simulink model "TST_EISGov_Governor"  (R2016b)
settings: Solver=FixedStepDiscrete  StartTime=0.0  StopTime=simTime  FixedStep=sampleTime  RelTol=1e-3
values from neighbouring files (symbols this model uses):
  testCase = 1    [initTST_EISGov_Governor_001.m]    (also in initTST_EISGov_Governor_002.m = 2; initTST_EISGov_Governor_003.m = 3; initTST_EISGov_Governor_004.m = 4; initTST_EISGov_Governor_005.m = 5)
libraries: simulink x43, UnitTest_Lib x36
(part 2 of 4)

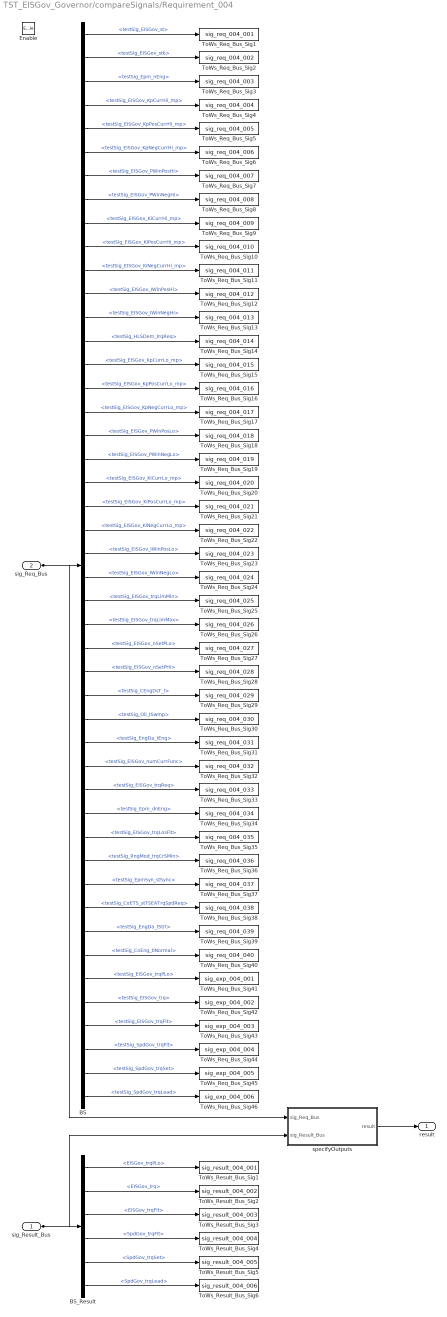
== system TST_EISGov_Governor/compareSignals/Requirement_004 ==
  sig_Result_Bus : Inport
  sig_Req_Bus : Inport  Port=2
  Enable : EnablePort
  BS : BusSelector  OutputSignals=testSig_EISGov_st,testSig_EISGov_st6,testSig_Epm_nEng,testSig_EISGov_KpCurrHi_mp,testSig_EISGov_KpPosCurrHi_mp,testSig_EISGov_KpNegCurrHi_mp,testSig_EISGov_PWinPosHi,testSig_EISGov_PWinNegHi,testSig_EISGov_KiCurrHi_mp,testSig_EISGov_KiPosCurrHi_mp,testSig_EISGov_KiNegCurrHi_mp,testSig_EISGov_IWinPosHi,testSig_EISGov_IWinNegHi,testSig_HLSDem_trqReq,testSig_EISGov_KpCurrLo_mp,testSig_EISGov_KpPosCurrLo_mp,testSig_EISGov_KpNegCurrLo_mp,testSig_EISGov_PWinPosLo,testSig_EISGov_PWinNegLo,testSig_EISGov_KiCurrLo_mp,testSig_EISGov_KiPosCurrLo_mp,testSig_EISGov_KiNegCurrLo_mp,testSig_EISGov_IWinPosLo,testSig_EISGov_IWinNegLo,testSig_EISGov_trqLimMin,testSig_EISGov_trqLimMax,testSig_EISGov_nSetPLo,testSig_EISGov_nSetPHi,testSig_CEngDsT_t,testSig_Oil_tSwmp,testSig_EngDa_tEng,testSig_EISGov_numCurrFunc,testSig_EISGov_trqReq,testSig_Epm_dnEng,testSig_EISGov_trqLosFlt,testSig_RngMod_trqCrSMin,testSig_EpmSyn_stSync,testSig_CoETS_stTSEATrqSpdReq,testSig_EngDa_tStrt,testSig_CoEng_tiNormal,testSig_EISGov_trqPLo,testSig_EISGov_trq,testSig_EISGov_trqFlt,testSig_SpdGov_trqFlt,testSig_SpdGov_trqSet,testSig_SpdGov_trqLead
  BS_Result : BusSelector  OutputSignals=EISGov_trqPLo,EISGov_trq,EISGov_trqFlt,SpdGov_trqFlt,SpdGov_trqSet,SpdGov_trqLead
  ToWs_Req_Bus_Sig1 : ToWorkspace  VariableName=sig_req_004_001  SaveFormat=Structure With Time
  ToWs_Req_Bus_Sig10 : ToWorkspace  VariableName=sig_req_004_010  SaveFormat=Structure With Time
  ToWs_Req_Bus_Sig11 : ToWorkspace  VariableName=sig_req_004_011  SaveFormat=Structure With Time
  ToWs_Req_Bus_Sig12 : ToWorkspace  VariableName=sig_req_004_012  SaveFormat=Structure With Time
  ToWs_Req_Bus_Sig13 : ToWorkspace  VariableName=sig_req_004_013  SaveFormat=Structure With Time
  ToWs_Req_Bus_Sig14 : ToWorkspace  VariableName=sig_req_004_014  SaveFormat=Structure With Time
  ToWs_Req_Bus_Sig15 : ToWorkspace  VariableName=sig_req_004_015  SaveFormat=Structure With Time
  ToWs_Req_Bus_Sig16 : ToWorkspace  VariableName=sig_req_004_016  SaveFormat=Structure With Time
  ToWs_Req_Bus_Sig17 : ToWorkspace  VariableName=sig_req_004_017  SaveFormat=Structure With Time
  ToWs_Req_Bus_Sig18 : ToWorkspace  VariableName=sig_req_004_018  SaveFormat=Structure With Time
  ToWs_Req_Bus_Sig19 : ToWorkspace  VariableName=sig_req_004_019  SaveFormat=Structure With Time
  ToWs_Req_Bus_Sig2 : ToWorkspace  VariableName=sig_req_004_002  SaveFormat=Structure With Time
  ToWs_Req_Bus_Sig20 : ToWorkspace  VariableName=sig_req_004_020  SaveFormat=Structure With Time
  ToWs_Req_Bus_Sig21 : ToWorkspace  VariableName=sig_req_004_021  SaveFormat=Structure With Time
  ToWs_Req_Bus_Sig22 : ToWorkspace  VariableName=sig_req_004_022  SaveFormat=Structure With Time
  ToWs_Req_Bus_Sig23 : ToWorkspace  VariableName=sig_req_004_023  SaveFormat=Structure With Time
  ToWs_Req_Bus_Sig24 : ToWorkspace  VariableName=sig_req_004_024  SaveFormat=Structure With Time
  ToWs_Req_Bus_Sig25 : ToWorkspace  VariableName=sig_req_004_025  SaveFormat=Structure With Time
  ToWs_Req_Bus_Sig26 : ToWorkspace  VariableName=sig_req_004_026  SaveFormat=Structure With Time
  ToWs_Req_Bus_Sig27 : ToWorkspace  VariableName=sig_req_004_027  SaveFormat=Structure With Time
  ToWs_Req_Bus_Sig28 : ToWorkspace  VariableName=sig_req_004_028  SaveFormat=Structure With Time
  ToWs_Req_Bus_Sig29 : ToWorkspace  VariableName=sig_req_004_029  SaveFormat=Structure With Time
  ToWs_Req_Bus_Sig3 : ToWorkspace  VariableName=sig_req_004_003  SaveFormat=Structure With Time
  ToWs_Req_Bus_Sig30 : ToWorkspace  VariableName=sig_req_004_030  SaveFormat=Structure With Time
  ToWs_Req_Bus_Sig31 : ToWorkspace  VariableName=sig_req_004_031  SaveFormat=Structure With Time
  ToWs_Req_Bus_Sig32 : ToWorkspace  VariableName=sig_req_004_032  SaveFormat=Structure With Time
  ToWs_Req_Bus_Sig33 : ToWorkspace  VariableName=sig_req_004_033  SaveFormat=Structure With Time
  ToWs_Req_Bus_Sig34 : ToWorkspace  VariableName=sig_req_004_034  SaveFormat=Structure With Time
  ToWs_Req_Bus_Sig35 : ToWorkspace  VariableName=sig_req_004_035  SaveFormat=Structure With Time
  ToWs_Req_Bus_Sig36 : ToWorkspace  VariableName=sig_req_004_036  SaveFormat=Structure With Time
  ToWs_Req_Bus_Sig37 : ToWorkspace  VariableName=sig_req_004_037  SaveFormat=Structure With Time
  ToWs_Req_Bus_Sig38 : ToWorkspace  VariableName=sig_req_004_038  SaveFormat=Structure With Time
  ToWs_Req_Bus_Sig39 : ToWorkspace  VariableName=sig_req_004_039  SaveFormat=Structure With Time
  ToWs_Req_Bus_Sig4 : ToWorkspace  VariableName=sig_req_004_004  SaveFormat=Structure With Time
  ToWs_Req_Bus_Sig40 : ToWorkspace  VariableName=sig_req_004_040  SaveFormat=Structure With Time
  ToWs_Req_Bus_Sig41 : ToWorkspace  VariableName=sig_exp_004_001  SaveFormat=Structure With Time
  ToWs_Req_Bus_Sig42 : ToWorkspace  VariableName=sig_exp_004_002  SaveFormat=Structure With Time
  ToWs_Req_Bus_Sig43 : ToWorkspace  VariableName=sig_exp_004_003  SaveFormat=Structure With Time
  ToWs_Req_Bus_Sig44 : ToWorkspace  VariableName=sig_exp_004_004  SaveFormat=Structure With Time
  ToWs_Req_Bus_Sig45 : ToWorkspace  VariableName=sig_exp_004_005  SaveFormat=Structure With Time
  ToWs_Req_Bus_Sig46 : ToWorkspace  VariableName=sig_exp_004_006  SaveFormat=Structure With Time
  ToWs_Req_Bus_Sig5 : ToWorkspace  VariableName=sig_req_004_005  SaveFormat=Structure With Time
  ToWs_Req_Bus_Sig6 : ToWorkspace  VariableName=sig_req_004_006  SaveFormat=Structure With Time
  ToWs_Req_Bus_Sig7 : ToWorkspace  VariableName=sig_req_004_007  SaveFormat=Structure With Time
  ToWs_Req_Bus_Sig8 : ToWorkspace  VariableName=sig_req_004_008  SaveFormat=Structure With Time
  ToWs_Req_Bus_Sig9 : ToWorkspace  VariableName=sig_req_004_009  SaveFormat=Structure With Time
  ToWs_Result_Bus_Sig1 : ToWorkspace  VariableName=sig_result_004_001  SaveFormat=Structure With Time
  ToWs_Result_Bus_Sig2 : ToWorkspace  VariableName=sig_result_004_002  SaveFormat=Structure With Time
  ToWs_Result_Bus_Sig3 : ToWorkspace  VariableName=sig_result_004_003  SaveFormat=Structure With Time
  ToWs_Result_Bus_Sig4 : ToWorkspace  VariableName=sig_result_004_004  SaveFormat=Structure With Time
  ToWs_Result_Bus_Sig5 : ToWorkspace  VariableName=sig_result_004_005  SaveFormat=Structure With Time
  ToWs_Result_Bus_Sig6 : ToWorkspace  VariableName=sig_result_004_006  SaveFormat=Structure With Time
  specifyOutputs : Subsystem
  result : Outport
  wires:
  sig_Req_Bus/1 -> BS/1, specifyOutputs/1(sig_Req_Bus)
  BS/1 -> ToWs_Req_Bus_Sig1/1  "<testSig_EISGov_st>"
  BS/2 -> ToWs_Req_Bus_Sig2/1  "<testSig_EISGov_st6>"
  BS/3 -> ToWs_Req_Bus_Sig3/1  "<testSig_Epm_nEng>"
  BS/4 -> ToWs_Req_Bus_Sig4/1  "<testSig_EISGov_KpCurrHi_mp>"
  BS/5 -> ToWs_Req_Bus_Sig5/1  "<testSig_EISGov_KpPosCurrHi_mp>"
  BS/6 -> ToWs_Req_Bus_Sig6/1  "<testSig_EISGov_KpNegCurrHi_mp>"
  BS/7 -> ToWs_Req_Bus_Sig7/1  "<testSig_EISGov_PWinPosHi>"
  BS/8 -> ToWs_Req_Bus_Sig8/1  "<testSig_EISGov_PWinNegHi>"
  BS/9 -> ToWs_Req_Bus_Sig9/1  "<testSig_EISGov_KiCurrHi_mp>"
  BS/10 -> ToWs_Req_Bus_Sig10/1  "<testSig_EISGov_KiPosCurrHi_mp>"
  BS/11 -> ToWs_Req_Bus_Sig11/1  "<testSig_EISGov_KiNegCurrHi_mp>"
  BS/12 -> ToWs_Req_Bus_Sig12/1  "<testSig_EISGov_IWinPosHi>"
  BS/13 -> ToWs_Req_Bus_Sig13/1  "<testSig_EISGov_IWinNegHi>"
  BS/14 -> ToWs_Req_Bus_Sig14/1  "<testSig_HLSDem_trqReq>"
  BS/15 -> ToWs_Req_Bus_Sig15/1  "<testSig_EISGov_KpCurrLo_mp>"
  BS/16 -> ToWs_Req_Bus_Sig16/1  "<testSig_EISGov_KpPosCurrLo_mp>"
  BS/17 -> ToWs_Req_Bus_Sig17/1  "<testSig_EISGov_KpNegCurrLo_mp>"
  BS/18 -> ToWs_Req_Bus_Sig18/1  "<testSig_EISGov_PWinPosLo>"
  BS/19 -> ToWs_Req_Bus_Sig19/1  "<testSig_EISGov_PWinNegLo>"
  BS/20 -> ToWs_Req_Bus_Sig20/1  "<testSig_EISGov_KiCurrLo_mp>"
  BS/21 -> ToWs_Req_Bus_Sig21/1  "<testSig_EISGov_KiPosCurrLo_mp>"
  BS/22 -> ToWs_Req_Bus_Sig22/1  "<testSig_EISGov_KiNegCurrLo_mp>"
  BS/23 -> ToWs_Req_Bus_Sig23/1  "<testSig_EISGov_IWinPosLo>"
  BS/24 -> ToWs_Req_Bus_Sig24/1  "<testSig_EISGov_IWinNegLo>"
  BS/25 -> ToWs_Req_Bus_Sig25/1  "<testSig_EISGov_trqLimMin>"
  BS/26 -> ToWs_Req_Bus_Sig26/1  "<testSig_EISGov_trqLimMax>"
  BS/27 -> ToWs_Req_Bus_Sig27/1  "<testSig_EISGov_nSetPLo>"
  BS/28 -> ToWs_Req_Bus_Sig28/1  "<testSig_EISGov_nSetPHi>"
  BS/29 -> ToWs_Req_Bus_Sig29/1  "<testSig_CEngDsT_t>"
  BS/30 -> ToWs_Req_Bus_Sig30/1  "<testSig_Oil_tSwmp>"
  BS/31 -> ToWs_Req_Bus_Sig31/1  "<testSig_EngDa_tEng>"
  BS/32 -> ToWs_Req_Bus_Sig32/1  "<testSig_EISGov_numCurrFunc>"
  BS/33 -> ToWs_Req_Bus_Sig33/1  "<testSig_EISGov_trqReq>"
  BS/34 -> ToWs_Req_Bus_Sig34/1  "<testSig_Epm_dnEng>"
  BS/35 -> ToWs_Req_Bus_Sig35/1  "<testSig_EISGov_trqLosFlt>"
  BS/36 -> ToWs_Req_Bus_Sig36/1  "<testSig_RngMod_trqCrSMin>"
  BS/37 -> ToWs_Req_Bus_Sig37/1  "<testSig_EpmSyn_stSync>"
  BS/38 -> ToWs_Req_Bus_Sig38/1  "<testSig_CoETS_stTSEATrqSpdReq>"
  BS/39 -> ToWs_Req_Bus_Sig39/1  "<testSig_EngDa_tStrt>"
  BS/40 -> ToWs_Req_Bus_Sig40/1  "<testSig_CoEng_tiNormal>"
  BS/41 -> ToWs_Req_Bus_Sig41/1  "<testSig_EISGov_trqPLo>"
  BS/42 -> ToWs_Req_Bus_Sig42/1  "<testSig_EISGov_trq>"
  BS/43 -> ToWs_Req_Bus_Sig43/1  "<testSig_EISGov_trqFlt>"
  BS/44 -> ToWs_Req_Bus_Sig44/1  "<testSig_SpdGov_trqFlt>"
  BS/45 -> ToWs_Req_Bus_Sig45/1  "<testSig_SpdGov_trqSet>"
  BS/46 -> ToWs_Req_Bus_Sig46/1  "<testSig_SpdGov_trqLead>"
  sig_Result_Bus/1 -> BS_Result/1, specifyOutputs/2(sig_Result_Bus)
  BS_Result/1 -> ToWs_Result_Bus_Sig1/1  "<EISGov_trqPLo>"
  BS_Result/2 -> ToWs_Result_Bus_Sig2/1  "<EISGov_trq>"
  BS_Result/3 -> ToWs_Result_Bus_Sig3/1  "<EISGov_trqFlt>"
  BS_Result/4 -> ToWs_Result_Bus_Sig4/1  "<SpdGov_trqFlt>"
  BS_Result/5 -> ToWs_Result_Bus_Sig5/1  "<SpdGov_trqSet>"
  BS_Result/6 -> ToWs_Result_Bus_Sig6/1  "<SpdGov_trqLead>"
  specifyOutputs/1(result) -> result/1

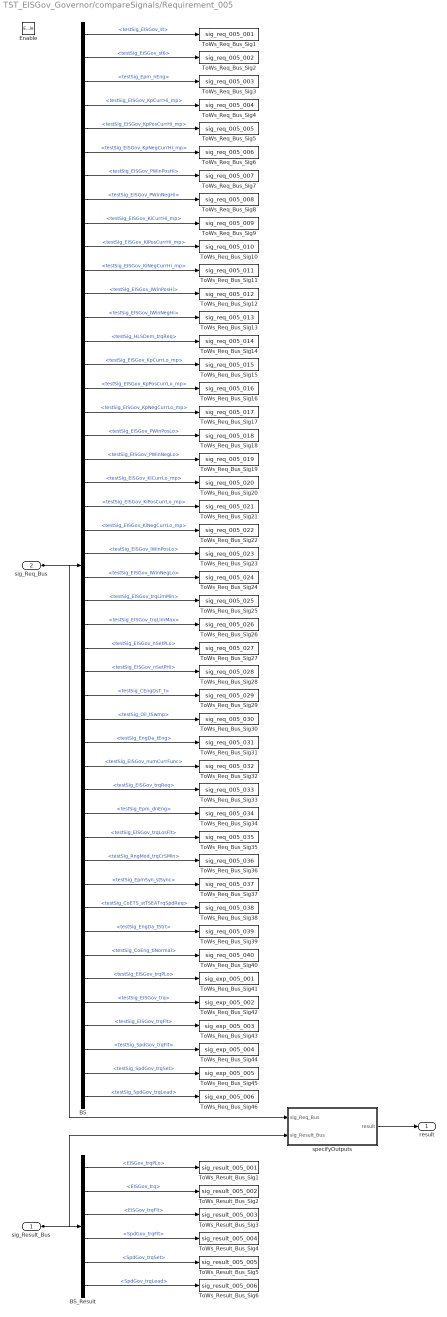
== system TST_EISGov_Governor/compareSignals/Requirement_005 ==
  sig_Result_Bus : Inport
  sig_Req_Bus : Inport  Port=2
  Enable : EnablePort
  BS : BusSelector  OutputSignals=testSig_EISGov_st,testSig_EISGov_st6,testSig_Epm_nEng,testSig_EISGov_KpCurrHi_mp,testSig_EISGov_KpPosCurrHi_mp,testSig_EISGov_KpNegCurrHi_mp,testSig_EISGov_PWinPosHi,testSig_EISGov_PWinNegHi,testSig_EISGov_KiCurrHi_mp,testSig_EISGov_KiPosCurrHi_mp,testSig_EISGov_KiNegCurrHi_mp,testSig_EISGov_IWinPosHi,testSig_EISGov_IWinNegHi,testSig_HLSDem_trqReq,testSig_EISGov_KpCurrLo_mp,testSig_EISGov_KpPosCurrLo_mp,testSig_EISGov_KpNegCurrLo_mp,testSig_EISGov_PWinPosLo,testSig_EISGov_PWinNegLo,testSig_EISGov_KiCurrLo_mp,testSig_EISGov_KiPosCurrLo_mp,testSig_EISGov_KiNegCurrLo_mp,testSig_EISGov_IWinPosLo,testSig_EISGov_IWinNegLo,testSig_EISGov_trqLimMin,testSig_EISGov_trqLimMax,testSig_EISGov_nSetPLo,testSig_EISGov_nSetPHi,testSig_CEngDsT_t,testSig_Oil_tSwmp,testSig_EngDa_tEng,testSig_EISGov_numCurrFunc,testSig_EISGov_trqReq,testSig_Epm_dnEng,testSig_EISGov_trqLosFlt,testSig_RngMod_trqCrSMin,testSig_EpmSyn_stSync,testSig_CoETS_stTSEATrqSpdReq,testSig_EngDa_tStrt,testSig_CoEng_tiNormal,testSig_EISGov_trqPLo,testSig_EISGov_trq,testSig_EISGov_trqFlt,testSig_SpdGov_trqFlt,testSig_SpdGov_trqSet,testSig_SpdGov_trqLead
  BS_Result : BusSelector  OutputSignals=EISGov_trqPLo,EISGov_trq,EISGov_trqFlt,SpdGov_trqFlt,SpdGov_trqSet,SpdGov_trqLead
  ToWs_Req_Bus_Sig1 : ToWorkspace  VariableName=sig_req_005_001  SaveFormat=Structure With Time
  ToWs_Req_Bus_Sig10 : ToWorkspace  VariableName=sig_req_005_010  SaveFormat=Structure With Time
  ToWs_Req_Bus_Sig11 : ToWorkspace  VariableName=sig_req_005_011  SaveFormat=Structure With Time
  ToWs_Req_Bus_Sig12 : ToWorkspace  VariableName=sig_req_005_012  SaveFormat=Structure With Time
  ToWs_Req_Bus_Sig13 : ToWorkspace  VariableName=sig_req_005_013  SaveFormat=Structure With Time
  ToWs_Req_Bus_Sig14 : ToWorkspace  VariableName=sig_req_005_014  SaveFormat=Structure With Time
  ToWs_Req_Bus_Sig15 : ToWorkspace  VariableName=sig_req_005_015  SaveFormat=Structure With Time
  ToWs_Req_Bus_Sig16 : ToWorkspace  VariableName=sig_req_005_016  SaveFormat=Structure With Time
  ToWs_Req_Bus_Sig17 : ToWorkspace  VariableName=sig_req_005_017  SaveFormat=Structure With Time
  ToWs_Req_Bus_Sig18 : ToWorkspace  VariableName=sig_req_005_018  SaveFormat=Structure With Time
  ToWs_Req_Bus_Sig19 : ToWorkspace  VariableName=sig_req_005_019  SaveFormat=Structure With Time
  ToWs_Req_Bus_Sig2 : ToWorkspace  VariableName=sig_req_005_002  SaveFormat=Structure With Time
  ToWs_Req_Bus_Sig20 : ToWorkspace  VariableName=sig_req_005_020  SaveFormat=Structure With Time
  ToWs_Req_Bus_Sig21 : ToWorkspace  VariableName=sig_req_005_021  SaveFormat=Structure With Time
  ToWs_Req_Bus_Sig22 : ToWorkspace  VariableName=sig_req_005_022  SaveFormat=Structure With Time
  ToWs_Req_Bus_Sig23 : ToWorkspace  VariableName=sig_req_005_023  SaveFormat=Structure With Time
  ToWs_Req_Bus_Sig24 : ToWorkspace  VariableName=sig_req_005_024  SaveFormat=Structure With Time
  ToWs_Req_Bus_Sig25 : ToWorkspace  VariableName=sig_req_005_025  SaveFormat=Structure With Time
  ToWs_Req_Bus_Sig26 : ToWorkspace  VariableName=sig_req_005_026  SaveFormat=Structure With Time
  ToWs_Req_Bus_Sig27 : ToWorkspace  VariableName=sig_req_005_027  SaveFormat=Structure With Time
  ToWs_Req_Bus_Sig28 : ToWorkspace  VariableName=sig_req_005_028  SaveFormat=Structure With Time
  ToWs_Req_Bus_Sig29 : ToWorkspace  VariableName=sig_req_005_029  SaveFormat=Structure With Time
  ToWs_Req_Bus_Sig3 : ToWorkspace  VariableName=sig_req_005_003  SaveFormat=Structure With Time
  ToWs_Req_Bus_Sig30 : ToWorkspace  VariableName=sig_req_005_030  SaveFormat=Structure With Time
  ToWs_Req_Bus_Sig31 : ToWorkspace  VariableName=sig_req_005_031  SaveFormat=Structure With Time
  ToWs_Req_Bus_Sig32 : ToWorkspace  VariableName=sig_req_005_032  SaveFormat=Structure With Time
  ToWs_Req_Bus_Sig33 : ToWorkspace  VariableName=sig_req_005_033  SaveFormat=Structure With Time
  ToWs_Req_Bus_Sig34 : ToWorkspace  VariableName=sig_req_005_034  SaveFormat=Structure With Time
  ToWs_Req_Bus_Sig35 : ToWorkspace  VariableName=sig_req_005_035  SaveFormat=Structure With Time
  ToWs_Req_Bus_Sig36 : ToWorkspace  VariableName=sig_req_005_036  SaveFormat=Structure With Time
  ToWs_Req_Bus_Sig37 : ToWorkspace  VariableName=sig_req_005_037  SaveFormat=Structure With Time
  ToWs_Req_Bus_Sig38 : ToWorkspace  VariableName=sig_req_005_038  SaveFormat=Structure With Time
  ToWs_Req_Bus_Sig39 : ToWorkspace  VariableName=sig_req_005_039  SaveFormat=Structure With Time
  ToWs_Req_Bus_Sig4 : ToWorkspace  VariableName=sig_req_005_004  SaveFormat=Structure With Time
  ToWs_Req_Bus_Sig40 : ToWorkspace  VariableName=sig_req_005_040  SaveFormat=Structure With Time
  ToWs_Req_Bus_Sig41 : ToWorkspace  VariableName=sig_exp_005_001  SaveFormat=Structure With Time
  ToWs_Req_Bus_Sig42 : ToWorkspace  VariableName=sig_exp_005_002  SaveFormat=Structure With Time
  ToWs_Req_Bus_Sig43 : ToWorkspace  VariableName=sig_exp_005_003  SaveFormat=Structure With Time
  ToWs_Req_Bus_Sig44 : ToWorkspace  VariableName=sig_exp_005_004  SaveFormat=Structure With Time
  ToWs_Req_Bus_Sig45 : ToWorkspace  VariableName=sig_exp_005_005  SaveFormat=Structure With Time
  ToWs_Req_Bus_Sig46 : ToWorkspace  VariableName=sig_exp_005_006  SaveFormat=Structure With Time
  ToWs_Req_Bus_Sig5 : ToWorkspace  VariableName=sig_req_005_005  SaveFormat=Structure With Time
  ToWs_Req_Bus_Sig6 : ToWorkspace  VariableName=sig_req_005_006  SaveFormat=Structure With Time
  ToWs_Req_Bus_Sig7 : ToWorkspace  VariableName=sig_req_005_007  SaveFormat=Structure With Time
  ToWs_Req_Bus_Sig8 : ToWorkspace  VariableName=sig_req_005_008  SaveFormat=Structure With Time
  ToWs_Req_Bus_Sig9 : ToWorkspace  VariableName=sig_req_005_009  SaveFormat=Structure With Time
  ToWs_Result_Bus_Sig1 : ToWorkspace  VariableName=sig_result_005_001  SaveFormat=Structure With Time
  ToWs_Result_Bus_Sig2 : ToWorkspace  VariableName=sig_result_005_002  SaveFormat=Structure With Time
  ToWs_Result_Bus_Sig3 : ToWorkspace  VariableName=sig_result_005_003  SaveFormat=Structure With Time
  ToWs_Result_Bus_Sig4 : ToWorkspace  VariableName=sig_result_005_004  SaveFormat=Structure With Time
  ToWs_Result_Bus_Sig5 : ToWorkspace  VariableName=sig_result_005_005  SaveFormat=Structure With Time
  ToWs_Result_Bus_Sig6 : ToWorkspace  VariableName=sig_result_005_006  SaveFormat=Structure With Time
  specifyOutputs : Subsystem
  result : Outport
  wires:
  sig_Req_Bus/1 -> BS/1, specifyOutputs/1(sig_Req_Bus)
  BS/1 -> ToWs_Req_Bus_Sig1/1  "<testSig_EISGov_st>"
  BS/2 -> ToWs_Req_Bus_Sig2/1  "<testSig_EISGov_st6>"
  BS/3 -> ToWs_Req_Bus_Sig3/1  "<testSig_Epm_nEng>"
  BS/4 -> ToWs_Req_Bus_Sig4/1  "<testSig_EISGov_KpCurrHi_mp>"
  BS/5 -> ToWs_Req_Bus_Sig5/1  "<testSig_EISGov_KpPosCurrHi_mp>"
  BS/6 -> ToWs_Req_Bus_Sig6/1  "<testSig_EISGov_KpNegCurrHi_mp>"
  BS/7 -> ToWs_Req_Bus_Sig7/1  "<testSig_EISGov_PWinPosHi>"
  BS/8 -> ToWs_Req_Bus_Sig8/1  "<testSig_EISGov_PWinNegHi>"
  BS/9 -> ToWs_Req_Bus_Sig9/1  "<testSig_EISGov_KiCurrHi_mp>"
  BS/10 -> ToWs_Req_Bus_Sig10/1  "<testSig_EISGov_KiPosCurrHi_mp>"
  BS/11 -> ToWs_Req_Bus_Sig11/1  "<testSig_EISGov_KiNegCurrHi_mp>"
  BS/12 -> ToWs_Req_Bus_Sig12/1  "<testSig_EISGov_IWinPosHi>"
  BS/13 -> ToWs_Req_Bus_Sig13/1  "<testSig_EISGov_IWinNegHi>"
  BS/14 -> ToWs_Req_Bus_Sig14/1  "<testSig_HLSDem_trqReq>"
  BS/15 -> ToWs_Req_Bus_Sig15/1  "<testSig_EISGov_KpCurrLo_mp>"
  BS/16 -> ToWs_Req_Bus_Sig16/1  "<testSig_EISGov_KpPosCurrLo_mp>"
  BS/17 -> ToWs_Req_Bus_Sig17/1  "<testSig_EISGov_KpNegCurrLo_mp>"
  BS/18 -> ToWs_Req_Bus_Sig18/1  "<testSig_EISGov_PWinPosLo>"
  BS/19 -> ToWs_Req_Bus_Sig19/1  "<testSig_EISGov_PWinNegLo>"
  BS/20 -> ToWs_Req_Bus_Sig20/1  "<testSig_EISGov_KiCurrLo_mp>"
  BS/21 -> ToWs_Req_Bus_Sig21/1  "<testSig_EISGov_KiPosCurrLo_mp>"
  BS/22 -> ToWs_Req_Bus_Sig22/1  "<testSig_EISGov_KiNegCurrLo_mp>"
  BS/23 -> ToWs_Req_Bus_Sig23/1  "<testSig_EISGov_IWinPosLo>"
  BS/24 -> ToWs_Req_Bus_Sig24/1  "<testSig_EISGov_IWinNegLo>"
  BS/25 -> ToWs_Req_Bus_Sig25/1  "<testSig_EISGov_trqLimMin>"
  BS/26 -> ToWs_Req_Bus_Sig26/1  "<testSig_EISGov_trqLimMax>"
  BS/27 -> ToWs_Req_Bus_Sig27/1  "<testSig_EISGov_nSetPLo>"
  BS/28 -> ToWs_Req_Bus_Sig28/1  "<testSig_EISGov_nSetPHi>"
  BS/29 -> ToWs_Req_Bus_Sig29/1  "<testSig_CEngDsT_t>"
  BS/30 -> ToWs_Req_Bus_Sig30/1  "<testSig_Oil_tSwmp>"
  BS/31 -> ToWs_Req_Bus_Sig31/1  "<testSig_EngDa_tEng>"
  BS/32 -> ToWs_Req_Bus_Sig32/1  "<testSig_EISGov_numCurrFunc>"
  BS/33 -> ToWs_Req_Bus_Sig33/1  "<testSig_EISGov_trqReq>"
  BS/34 -> ToWs_Req_Bus_Sig34/1  "<testSig_Epm_dnEng>"
  BS/35 -> ToWs_Req_Bus_Sig35/1  "<testSig_EISGov_trqLosFlt>"
  BS/36 -> ToWs_Req_Bus_Sig36/1  "<testSig_RngMod_trqCrSMin>"
  BS/37 -> ToWs_Req_Bus_Sig37/1  "<testSig_EpmSyn_stSync>"
  BS/38 -> ToWs_Req_Bus_Sig38/1  "<testSig_CoETS_stTSEATrqSpdReq>"
  BS/39 -> ToWs_Req_Bus_Sig39/1  "<testSig_EngDa_tStrt>"
  BS/40 -> ToWs_Req_Bus_Sig40/1  "<testSig_CoEng_tiNormal>"
  BS/41 -> ToWs_Req_Bus_Sig41/1  "<testSig_EISGov_trqPLo>"
  BS/42 -> ToWs_Req_Bus_Sig42/1  "<testSig_EISGov_trq>"
  BS/43 -> ToWs_Req_Bus_Sig43/1  "<testSig_EISGov_trqFlt>"
  BS/44 -> ToWs_Req_Bus_Sig44/1  "<testSig_SpdGov_trqFlt>"
  BS/45 -> ToWs_Req_Bus_Sig45/1  "<testSig_SpdGov_trqSet>"
  BS/46 -> ToWs_Req_Bus_Sig46/1  "<testSig_SpdGov_trqLead>"
  sig_Result_Bus/1 -> BS_Result/1, specifyOutputs/2(sig_Result_Bus)
  BS_Result/1 -> ToWs_Result_Bus_Sig1/1  "<EISGov_trqPLo>"
  BS_Result/2 -> ToWs_Result_Bus_Sig2/1  "<EISGov_trq>"
  BS_Result/3 -> ToWs_Result_Bus_Sig3/1  "<EISGov_trqFlt>"
  BS_Result/4 -> ToWs_Result_Bus_Sig4/1  "<SpdGov_trqFlt>"
  BS_Result/5 -> ToWs_Result_Bus_Sig5/1  "<SpdGov_trqSet>"
  BS_Result/6 -> ToWs_Result_Bus_Sig6/1  "<SpdGov_trqLead>"
  specifyOutputs/1(result) -> result/1

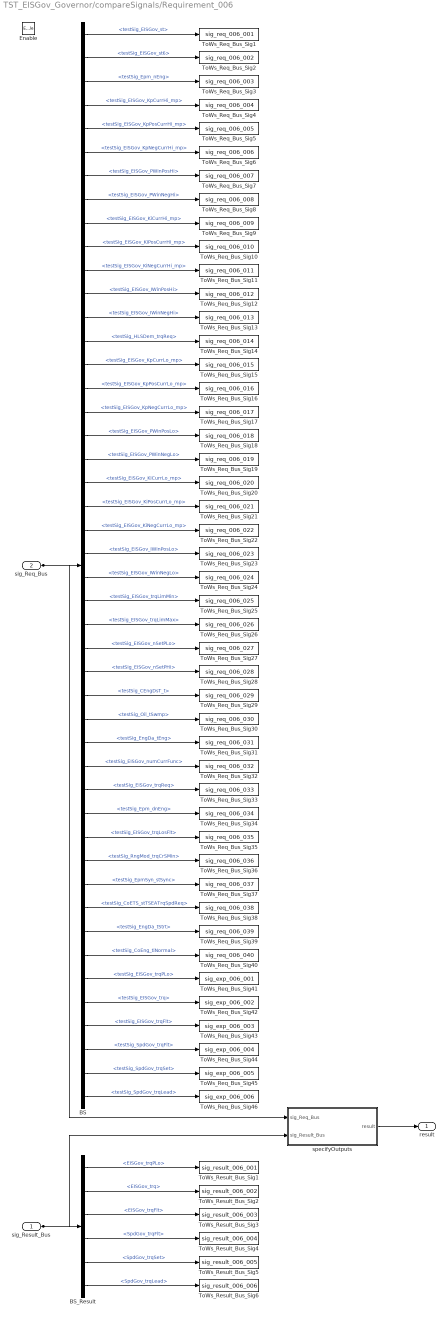
== system TST_EISGov_Governor/compareSignals/Requirement_006 ==
  sig_Result_Bus : Inport
  sig_Req_Bus : Inport  Port=2
  Enable : EnablePort
  BS : BusSelector  OutputSignals=testSig_EISGov_st,testSig_EISGov_st6,testSig_Epm_nEng,testSig_EISGov_KpCurrHi_mp,testSig_EISGov_KpPosCurrHi_mp,testSig_EISGov_KpNegCurrHi_mp,testSig_EISGov_PWinPosHi,testSig_EISGov_PWinNegHi,testSig_EISGov_KiCurrHi_mp,testSig_EISGov_KiPosCurrHi_mp,testSig_EISGov_KiNegCurrHi_mp,testSig_EISGov_IWinPosHi,testSig_EISGov_IWinNegHi,testSig_HLSDem_trqReq,testSig_EISGov_KpCurrLo_mp,testSig_EISGov_KpPosCurrLo_mp,testSig_EISGov_KpNegCurrLo_mp,testSig_EISGov_PWinPosLo,testSig_EISGov_PWinNegLo,testSig_EISGov_KiCurrLo_mp,testSig_EISGov_KiPosCurrLo_mp,testSig_EISGov_KiNegCurrLo_mp,testSig_EISGov_IWinPosLo,testSig_EISGov_IWinNegLo,testSig_EISGov_trqLimMin,testSig_EISGov_trqLimMax,testSig_EISGov_nSetPLo,testSig_EISGov_nSetPHi,testSig_CEngDsT_t,testSig_Oil_tSwmp,testSig_EngDa_tEng,testSig_EISGov_numCurrFunc,testSig_EISGov_trqReq,testSig_Epm_dnEng,testSig_EISGov_trqLosFlt,testSig_RngMod_trqCrSMin,testSig_EpmSyn_stSync,testSig_CoETS_stTSEATrqSpdReq,testSig_EngDa_tStrt,testSig_CoEng_tiNormal,testSig_EISGov_trqPLo,testSig_EISGov_trq,testSig_EISGov_trqFlt,testSig_SpdGov_trqFlt,testSig_SpdGov_trqSet,testSig_SpdGov_trqLead
  BS_Result : BusSelector  OutputSignals=EISGov_trqPLo,EISGov_trq,EISGov_trqFlt,SpdGov_trqFlt,SpdGov_trqSet,SpdGov_trqLead
  ToWs_Req_Bus_Sig1 : ToWorkspace  VariableName=sig_req_006_001  SaveFormat=Structure With Time
  ToWs_Req_Bus_Sig10 : ToWorkspace  VariableName=sig_req_006_010  SaveFormat=Structure With Time
  ToWs_Req_Bus_Sig11 : ToWorkspace  VariableName=sig_req_006_011  SaveFormat=Structure With Time
  ToWs_Req_Bus_Sig12 : ToWorkspace  VariableName=sig_req_006_012  SaveFormat=Structure With Time
  ToWs_Req_Bus_Sig13 : ToWorkspace  VariableName=sig_req_006_013  SaveFormat=Structure With Time
  ToWs_Req_Bus_Sig14 : ToWorkspace  VariableName=sig_req_006_014  SaveFormat=Structure With Time
  ToWs_Req_Bus_Sig15 : ToWorkspace  VariableName=sig_req_006_015  SaveFormat=Structure With Time
  ToWs_Req_Bus_Sig16 : ToWorkspace  VariableName=sig_req_006_016  SaveFormat=Structure With Time
  ToWs_Req_Bus_Sig17 : ToWorkspace  VariableName=sig_req_006_017  SaveFormat=Structure With Time
  ToWs_Req_Bus_Sig18 : ToWorkspace  VariableName=sig_req_006_018  SaveFormat=Structure With Time
  ToWs_Req_Bus_Sig19 : ToWorkspace  VariableName=sig_req_006_019  SaveFormat=Structure With Time
  ToWs_Req_Bus_Sig2 : ToWorkspace  VariableName=sig_req_006_002  SaveFormat=Structure With Time
  ToWs_Req_Bus_Sig20 : ToWorkspace  VariableName=sig_req_006_020  SaveFormat=Structure With Time
  ToWs_Req_Bus_Sig21 : ToWorkspace  VariableName=sig_req_006_021  SaveFormat=Structure With Time
  ToWs_Req_Bus_Sig22 : ToWorkspace  VariableName=sig_req_006_022  SaveFormat=Structure With Time
  ToWs_Req_Bus_Sig23 : ToWorkspace  VariableName=sig_req_006_023  SaveFormat=Structure With Time
  ToWs_Req_Bus_Sig24 : ToWorkspace  VariableName=sig_req_006_024  SaveFormat=Structure With Time
  ToWs_Req_Bus_Sig25 : ToWorkspace  VariableName=sig_req_006_025  SaveFormat=Structure With Time
  ToWs_Req_Bus_Sig26 : ToWorkspace  VariableName=sig_req_006_026  SaveFormat=Structure With Time
  ToWs_Req_Bus_Sig27 : ToWorkspace  VariableName=sig_req_006_027  SaveFormat=Structure With Time
  ToWs_Req_Bus_Sig28 : ToWorkspace  VariableName=sig_req_006_028  SaveFormat=Structure With Time
  ToWs_Req_Bus_Sig29 : ToWorkspace  VariableName=sig_req_006_029  SaveFormat=Structure With Time
  ToWs_Req_Bus_Sig3 : ToWorkspace  VariableName=sig_req_006_003  SaveFormat=Structure With Time
  ToWs_Req_Bus_Sig30 : ToWorkspace  VariableName=sig_req_006_030  SaveFormat=Structure With Time
  ToWs_Req_Bus_Sig31 : ToWorkspace  VariableName=sig_req_006_031  SaveFormat=Structure With Time
  ToWs_Req_Bus_Sig32 : ToWorkspace  VariableName=sig_req_006_032  SaveFormat=Structure With Time
  ToWs_Req_Bus_Sig33 : ToWorkspace  VariableName=sig_req_006_033  SaveFormat=Structure With Time
  ToWs_Req_Bus_Sig34 : ToWorkspace  VariableName=sig_req_006_034  SaveFormat=Structure With Time
  ToWs_Req_Bus_Sig35 : ToWorkspace  VariableName=sig_req_006_035  SaveFormat=Structure With Time
  ToWs_Req_Bus_Sig36 : ToWorkspace  VariableName=sig_req_006_036  SaveFormat=Structure With Time
  ToWs_Req_Bus_Sig37 : ToWorkspace  VariableName=sig_req_006_037  SaveFormat=Structure With Time
  ToWs_Req_Bus_Sig38 : ToWorkspace  VariableName=sig_req_006_038  SaveFormat=Structure With Time
  ToWs_Req_Bus_Sig39 : ToWorkspace  VariableName=sig_req_006_039  SaveFormat=Structure With Time
  ToWs_Req_Bus_Sig4 : ToWorkspace  VariableName=sig_req_006_004  SaveFormat=Structure With Time
  ToWs_Req_Bus_Sig40 : ToWorkspace  VariableName=sig_req_006_040  SaveFormat=Structure With Time
  ToWs_Req_Bus_Sig41 : ToWorkspace  VariableName=sig_exp_006_001  SaveFormat=Structure With Time
  ToWs_Req_Bus_Sig42 : ToWorkspace  VariableName=sig_exp_006_002  SaveFormat=Structure With Time
  ToWs_Req_Bus_Sig43 : ToWorkspace  VariableName=sig_exp_006_003  SaveFormat=Structure With Time
  ToWs_Req_Bus_Sig44 : ToWorkspace  VariableName=sig_exp_006_004  SaveFormat=Structure With Time
  ToWs_Req_Bus_Sig45 : ToWorkspace  VariableName=sig_exp_006_005  SaveFormat=Structure With Time
  ToWs_Req_Bus_Sig46 : ToWorkspace  VariableName=sig_exp_006_006  SaveFormat=Structure With Time
  ToWs_Req_Bus_Sig5 : ToWorkspace  VariableName=sig_req_006_005  SaveFormat=Structure With Time
  ToWs_Req_Bus_Sig6 : ToWorkspace  VariableName=sig_req_006_006  SaveFormat=Structure With Time
  ToWs_Req_Bus_Sig7 : ToWorkspace  VariableName=sig_req_006_007  SaveFormat=Structure With Time
  ToWs_Req_Bus_Sig8 : ToWorkspace  VariableName=sig_req_006_008  SaveFormat=Structure With Time
  ToWs_Req_Bus_Sig9 : ToWorkspace  VariableName=sig_req_006_009  SaveFormat=Structure With Time
  ToWs_Result_Bus_Sig1 : ToWorkspace  VariableName=sig_result_006_001  SaveFormat=Structure With Time
  ToWs_Result_Bus_Sig2 : ToWorkspace  VariableName=sig_result_006_002  SaveFormat=Structure With Time
  ToWs_Result_Bus_Sig3 : ToWorkspace  VariableName=sig_result_006_003  SaveFormat=Structure With Time
  ToWs_Result_Bus_Sig4 : ToWorkspace  VariableName=sig_result_006_004  SaveFormat=Structure With Time
  ToWs_Result_Bus_Sig5 : ToWorkspace  VariableName=sig_result_006_005  SaveFormat=Structure With Time
  ToWs_Result_Bus_Sig6 : ToWorkspace  VariableName=sig_result_006_006  SaveFormat=Structure With Time
  specifyOutputs : Subsystem
  result : Outport
  wires:
  sig_Req_Bus/1 -> BS/1, specifyOutputs/1(sig_Req_Bus)
  BS/1 -> ToWs_Req_Bus_Sig1/1  "<testSig_EISGov_st>"
  BS/2 -> ToWs_Req_Bus_Sig2/1  "<testSig_EISGov_st6>"
  BS/3 -> ToWs_Req_Bus_Sig3/1  "<testSig_Epm_nEng>"
  BS/4 -> ToWs_Req_Bus_Sig4/1  "<testSig_EISGov_KpCurrHi_mp>"
  BS/5 -> ToWs_Req_Bus_Sig5/1  "<testSig_EISGov_KpPosCurrHi_mp>"
  BS/6 -> ToWs_Req_Bus_Sig6/1  "<testSig_EISGov_KpNegCurrHi_mp>"
  BS/7 -> ToWs_Req_Bus_Sig7/1  "<testSig_EISGov_PWinPosHi>"
  BS/8 -> ToWs_Req_Bus_Sig8/1  "<testSig_EISGov_PWinNegHi>"
  BS/9 -> ToWs_Req_Bus_Sig9/1  "<testSig_EISGov_KiCurrHi_mp>"
  BS/10 -> ToWs_Req_Bus_Sig10/1  "<testSig_EISGov_KiPosCurrHi_mp>"
  BS/11 -> ToWs_Req_Bus_Sig11/1  "<testSig_EISGov_KiNegCurrHi_mp>"
  BS/12 -> ToWs_Req_Bus_Sig12/1  "<testSig_EISGov_IWinPosHi>"
  BS/13 -> ToWs_Req_Bus_Sig13/1  "<testSig_EISGov_IWinNegHi>"
  BS/14 -> ToWs_Req_Bus_Sig14/1  "<testSig_HLSDem_trqReq>"
  BS/15 -> ToWs_Req_Bus_Sig15/1  "<testSig_EISGov_KpCurrLo_mp>"
  BS/16 -> ToWs_Req_Bus_Sig16/1  "<testSig_EISGov_KpPosCurrLo_mp>"
  BS/17 -> ToWs_Req_Bus_Sig17/1  "<testSig_EISGov_KpNegCurrLo_mp>"
  BS/18 -> ToWs_Req_Bus_Sig18/1  "<testSig_EISGov_PWinPosLo>"
  BS/19 -> ToWs_Req_Bus_Sig19/1  "<testSig_EISGov_PWinNegLo>"
  BS/20 -> ToWs_Req_Bus_Sig20/1  "<testSig_EISGov_KiCurrLo_mp>"
  BS/21 -> ToWs_Req_Bus_Sig21/1  "<testSig_EISGov_KiPosCurrLo_mp>"
  BS/22 -> ToWs_Req_Bus_Sig22/1  "<testSig_EISGov_KiNegCurrLo_mp>"
  BS/23 -> ToWs_Req_Bus_Sig23/1  "<testSig_EISGov_IWinPosLo>"
  BS/24 -> ToWs_Req_Bus_Sig24/1  "<testSig_EISGov_IWinNegLo>"
  BS/25 -> ToWs_Req_Bus_Sig25/1  "<testSig_EISGov_trqLimMin>"
  BS/26 -> ToWs_Req_Bus_Sig26/1  "<testSig_EISGov_trqLimMax>"
  BS/27 -> ToWs_Req_Bus_Sig27/1  "<testSig_EISGov_nSetPLo>"
  BS/28 -> ToWs_Req_Bus_Sig28/1  "<testSig_EISGov_nSetPHi>"
  BS/29 -> ToWs_Req_Bus_Sig29/1  "<testSig_CEngDsT_t>"
  BS/30 -> ToWs_Req_Bus_Sig30/1  "<testSig_Oil_tSwmp>"
  BS/31 -> ToWs_Req_Bus_Sig31/1  "<testSig_EngDa_tEng>"
  BS/32 -> ToWs_Req_Bus_Sig32/1  "<testSig_EISGov_numCurrFunc>"
  BS/33 -> ToWs_Req_Bus_Sig33/1  "<testSig_EISGov_trqReq>"
  BS/34 -> ToWs_Req_Bus_Sig34/1  "<testSig_Epm_dnEng>"
  BS/35 -> ToWs_Req_Bus_Sig35/1  "<testSig_EISGov_trqLosFlt>"
  BS/36 -> ToWs_Req_Bus_Sig36/1  "<testSig_RngMod_trqCrSMin>"
  BS/37 -> ToWs_Req_Bus_Sig37/1  "<testSig_EpmSyn_stSync>"
  BS/38 -> ToWs_Req_Bus_Sig38/1  "<testSig_CoETS_stTSEATrqSpdReq>"
  BS/39 -> ToWs_Req_Bus_Sig39/1  "<testSig_EngDa_tStrt>"
  BS/40 -> ToWs_Req_Bus_Sig40/1  "<testSig_CoEng_tiNormal>"
  BS/41 -> ToWs_Req_Bus_Sig41/1  "<testSig_EISGov_trqPLo>"
  BS/42 -> ToWs_Req_Bus_Sig42/1  "<testSig_EISGov_trq>"
  BS/43 -> ToWs_Req_Bus_Sig43/1  "<testSig_EISGov_trqFlt>"
  BS/44 -> ToWs_Req_Bus_Sig44/1  "<testSig_SpdGov_trqFlt>"
  BS/45 -> ToWs_Req_Bus_Sig45/1  "<testSig_SpdGov_trqSet>"
  BS/46 -> ToWs_Req_Bus_Sig46/1  "<testSig_SpdGov_trqLead>"
  sig_Result_Bus/1 -> BS_Result/1, specifyOutputs/2(sig_Result_Bus)
  BS_Result/1 -> ToWs_Result_Bus_Sig1/1  "<EISGov_trqPLo>"
  BS_Result/2 -> ToWs_Result_Bus_Sig2/1  "<EISGov_trq>"
  BS_Result/3 -> ToWs_Result_Bus_Sig3/1  "<EISGov_trqFlt>"
  BS_Result/4 -> ToWs_Result_Bus_Sig4/1  "<SpdGov_trqFlt>"
  BS_Result/5 -> ToWs_Result_Bus_Sig5/1  "<SpdGov_trqSet>"
  BS_Result/6 -> ToWs_Result_Bus_Sig6/1  "<SpdGov_trqLead>"
  specifyOutputs/1(result) -> result/1

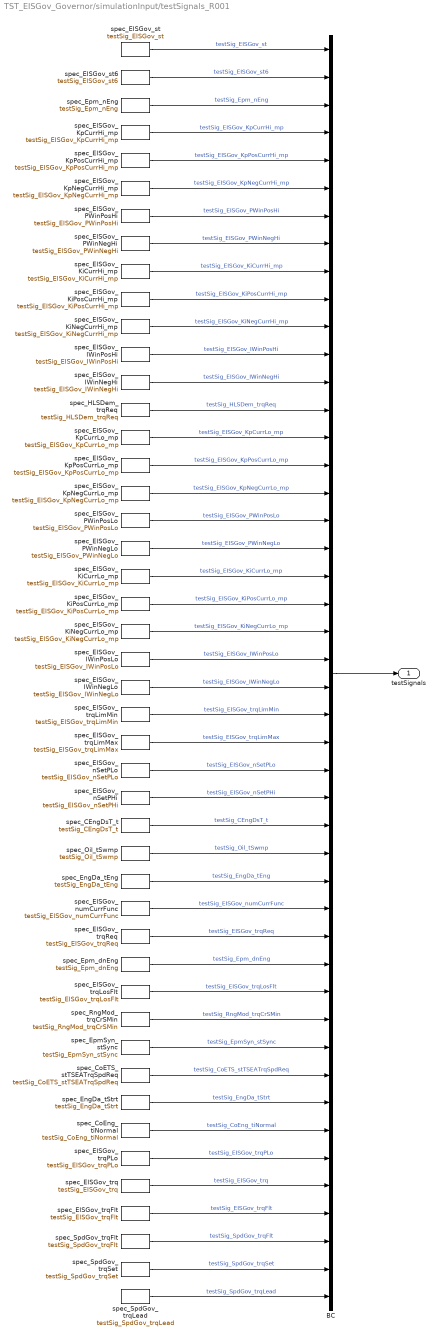
== system TST_EISGov_Governor/simulationInput/testSignals_R001 ==
  BC : BusCreator  Inputs=46
  spec_CEngDsT_t : FromWorkspace  VariableName=testSig_CEngDsT_t  Interpolate=off  OutputAfterFinalValue=Holding final value
  spec_CoETS_stTSEATrqSpdReq : FromWorkspace  VariableName=testSig_CoETS_stTSEATrqSpdReq  Interpolate=off  OutputAfterFinalValue=Holding final value
  spec_CoEng_tiNormal : FromWorkspace  VariableName=testSig_CoEng_tiNormal  Interpolate=off  OutputAfterFinalValue=Holding final value
  spec_EISGov_IWinNegHi : FromWorkspace  VariableName=testSig_EISGov_IWinNegHi  Interpolate=off  OutputAfterFinalValue=Holding final value
  spec_EISGov_IWinNegLo : FromWorkspace  VariableName=testSig_EISGov_IWinNegLo  Interpolate=off  OutputAfterFinalValue=Holding final value
  spec_EISGov_IWinPosHi : FromWorkspace  VariableName=testSig_EISGov_IWinPosHi  Interpolate=off  OutputAfterFinalValue=Holding final value
  spec_EISGov_IWinPosLo : FromWorkspace  VariableName=testSig_EISGov_IWinPosLo  Interpolate=off  OutputAfterFinalValue=Holding final value
  spec_EISGov_KiCurrHi_mp : FromWorkspace  VariableName=testSig_EISGov_KiCurrHi_mp  Interpolate=off  OutputAfterFinalValue=Holding final value
  spec_EISGov_KiCurrLo_mp : FromWorkspace  VariableName=testSig_EISGov_KiCurrLo_mp  Interpolate=off  OutputAfterFinalValue=Holding final value
  spec_EISGov_KiNegCurrHi_mp : FromWorkspace  VariableName=testSig_EISGov_KiNegCurrHi_mp  Interpolate=off  OutputAfterFinalValue=Holding final value
  spec_EISGov_KiNegCurrLo_mp : FromWorkspace  VariableName=testSig_EISGov_KiNegCurrLo_mp  Interpolate=off  OutputAfterFinalValue=Holding final value
  spec_EISGov_KiPosCurrHi_mp : FromWorkspace  VariableName=testSig_EISGov_KiPosCurrHi_mp  Interpolate=off  OutputAfterFinalValue=Holding final value
  spec_EISGov_KiPosCurrLo_mp : FromWorkspace  VariableName=testSig_EISGov_KiPosCurrLo_mp  Interpolate=off  OutputAfterFinalValue=Holding final value
  spec_EISGov_KpCurrHi_mp : FromWorkspace  VariableName=testSig_EISGov_KpCurrHi_mp  Interpolate=off  OutputAfterFinalValue=Holding final value
  spec_EISGov_KpCurrLo_mp : FromWorkspace  VariableName=testSig_EISGov_KpCurrLo_mp  Interpolate=off  OutputAfterFinalValue=Holding final value
  spec_EISGov_KpNegCurrHi_mp : FromWorkspace  VariableName=testSig_EISGov_KpNegCurrHi_mp  Interpolate=off  OutputAfterFinalValue=Holding final value
  spec_EISGov_KpNegCurrLo_mp : FromWorkspace  VariableName=testSig_EISGov_KpNegCurrLo_mp  Interpolate=off  OutputAfterFinalValue=Holding final value
  spec_EISGov_KpPosCurrHi_mp : FromWorkspace  VariableName=testSig_EISGov_KpPosCurrHi_mp  Interpolate=off  OutputAfterFinalValue=Holding final value
  spec_EISGov_KpPosCurrLo_mp : FromWorkspace  VariableName=testSig_EISGov_KpPosCurrLo_mp  Interpolate=off  OutputAfterFinalValue=Holding final value
  spec_EISGov_PWinNegHi : FromWorkspace  VariableName=testSig_EISGov_PWinNegHi  Interpolate=off  OutputAfterFinalValue=Holding final value
  spec_EISGov_PWinNegLo : FromWorkspace  VariableName=testSig_EISGov_PWinNegLo  Interpolate=off  OutputAfterFinalValue=Holding final value
  spec_EISGov_PWinPosHi : FromWorkspace  VariableName=testSig_EISGov_PWinPosHi  Interpolate=off  OutputAfterFinalValue=Holding final value
  spec_EISGov_PWinPosLo : FromWorkspace  VariableName=testSig_EISGov_PWinPosLo  Interpolate=off  OutputAfterFinalValue=Holding final value
  spec_EISGov_nSetPHi : FromWorkspace  VariableName=testSig_EISGov_nSetPHi  Interpolate=off  OutputAfterFinalValue=Holding final value
  spec_EISGov_nSetPLo : FromWorkspace  VariableName=testSig_EISGov_nSetPLo  Interpolate=off  OutputAfterFinalValue=Holding final value
  spec_EISGov_numCurrFunc : FromWorkspace  VariableName=testSig_EISGov_numCurrFunc  Interpolate=off  OutputAfterFinalValue=Holding final value
  spec_EISGov_st : FromWorkspace  VariableName=testSig_EISGov_st  Interpolate=off  OutputAfterFinalValue=Holding final value
  spec_EISGov_st6 : FromWorkspace  VariableName=testSig_EISGov_st6  Interpolate=off  OutputAfterFinalValue=Holding final value
  spec_EISGov_trq : FromWorkspace  VariableName=testSig_EISGov_trq  Interpolate=off  OutputAfterFinalValue=Holding final value
  spec_EISGov_trqFlt : FromWorkspace  VariableName=testSig_EISGov_trqFlt  Interpolate=off  OutputAfterFinalValue=Holding final value
  spec_EISGov_trqLimMax : FromWorkspace  VariableName=testSig_EISGov_trqLimMax  Interpolate=off  OutputAfterFinalValue=Holding final value
  spec_EISGov_trqLimMin : FromWorkspace  VariableName=testSig_EISGov_trqLimMin  Interpolate=off  OutputAfterFinalValue=Holding final value
  spec_EISGov_trqLosFlt : FromWorkspace  VariableName=testSig_EISGov_trqLosFlt  Interpolate=off  OutputAfterFinalValue=Holding final value
  spec_EISGov_trqPLo : FromWorkspace  VariableName=testSig_EISGov_trqPLo  Interpolate=off  OutputAfterFinalValue=Holding final value
  spec_EISGov_trqReq : FromWorkspace  VariableName=testSig_EISGov_trqReq  Interpolate=off  OutputAfterFinalValue=Holding final value
  spec_EngDa_tEng : FromWorkspace  VariableName=testSig_EngDa_tEng  Interpolate=off  OutputAfterFinalValue=Holding final value
  spec_EngDa_tStrt : FromWorkspace  VariableName=testSig_EngDa_tStrt  Interpolate=off  OutputAfterFinalValue=Holding final value
  spec_EpmSyn_stSync : FromWorkspace  VariableName=testSig_EpmSyn_stSync  Interpolate=off  OutputAfterFinalValue=Holding final value
  spec_Epm_dnEng : FromWorkspace  VariableName=testSig_Epm_dnEng  Interpolate=off  OutputAfterFinalValue=Holding final value
  spec_Epm_nEng : FromWorkspace  VariableName=testSig_Epm_nEng  Interpolate=off  OutputAfterFinalValue=Holding final value
  spec_HLSDem_trqReq : FromWorkspace  VariableName=testSig_HLSDem_trqReq  Interpolate=off  OutputAfterFinalValue=Holding final value
  spec_Oil_tSwmp : FromWorkspace  VariableName=testSig_Oil_tSwmp  Interpolate=off  OutputAfterFinalValue=Holding final value
  spec_RngMod_trqCrSMin : FromWorkspace  VariableName=testSig_RngMod_trqCrSMin  Interpolate=off  OutputAfterFinalValue=Holding final value
  spec_SpdGov_trqFlt : FromWorkspace  VariableName=testSig_SpdGov_trqFlt  Interpolate=off  OutputAfterFinalValue=Holding final value
  spec_SpdGov_trqLead : FromWorkspace  VariableName=testSig_SpdGov_trqLead  Interpolate=off  OutputAfterFinalValue=Holding final value
  spec_SpdGov_trqSet : FromWorkspace  VariableName=testSig_SpdGov_trqSet  Interpolate=off  OutputAfterFinalValue=Holding final value
  testSignals : Outport
  wires:
  BC/1 -> testSignals/1
  spec_EISGov_st/1 -> BC/1  "testSig_EISGov_st"
  spec_EISGov_st6/1 -> BC/2  "testSig_EISGov_st6"
  spec_Epm_nEng/1 -> BC/3  "testSig_Epm_nEng"
  spec_EISGov_KpCurrHi_mp/1 -> BC/4  "testSig_EISGov_KpCurrHi_mp"
  spec_EISGov_KpPosCurrHi_mp/1 -> BC/5  "testSig_EISGov_KpPosCurrHi_mp"
  spec_EISGov_KpNegCurrHi_mp/1 -> BC/6  "testSig_EISGov_KpNegCurrHi_mp"
  spec_EISGov_PWinPosHi/1 -> BC/7  "testSig_EISGov_PWinPosHi"
  spec_EISGov_PWinNegHi/1 -> BC/8  "testSig_EISGov_PWinNegHi"
  spec_EISGov_KiCurrHi_mp/1 -> BC/9  "testSig_EISGov_KiCurrHi_mp"
  spec_EISGov_KiPosCurrHi_mp/1 -> BC/10  "testSig_EISGov_KiPosCurrHi_mp"
  spec_EISGov_KiNegCurrHi_mp/1 -> BC/11  "testSig_EISGov_KiNegCurrHi_mp"
  spec_EISGov_IWinPosHi/1 -> BC/12  "testSig_EISGov_IWinPosHi"
  spec_EISGov_IWinNegHi/1 -> BC/13  "testSig_EISGov_IWinNegHi"
  spec_HLSDem_trqReq/1 -> BC/14  "testSig_HLSDem_trqReq"
  spec_EISGov_KpCurrLo_mp/1 -> BC/15  "testSig_EISGov_KpCurrLo_mp"
  spec_EISGov_KpPosCurrLo_mp/1 -> BC/16  "testSig_EISGov_KpPosCurrLo_mp"
  spec_EISGov_KpNegCurrLo_mp/1 -> BC/17  "testSig_EISGov_KpNegCurrLo_mp"
  spec_EISGov_PWinPosLo/1 -> BC/18  "testSig_EISGov_PWinPosLo"
  spec_EISGov_PWinNegLo/1 -> BC/19  "testSig_EISGov_PWinNegLo"
  spec_EISGov_KiCurrLo_mp/1 -> BC/20  "testSig_EISGov_KiCurrLo_mp"
  spec_EISGov_KiPosCurrLo_mp/1 -> BC/21  "testSig_EISGov_KiPosCurrLo_mp"
  spec_EISGov_KiNegCurrLo_mp/1 -> BC/22  "testSig_EISGov_KiNegCurrLo_mp"
  spec_EISGov_IWinPosLo/1 -> BC/23  "testSig_EISGov_IWinPosLo"
  spec_EISGov_IWinNegLo/1 -> BC/24  "testSig_EISGov_IWinNegLo"
  spec_EISGov_trqLimMin/1 -> BC/25  "testSig_EISGov_trqLimMin"
  spec_EISGov_trqLimMax/1 -> BC/26  "testSig_EISGov_trqLimMax"
  spec_EISGov_nSetPLo/1 -> BC/27  "testSig_EISGov_nSetPLo"
  spec_EISGov_nSetPHi/1 -> BC/28  "testSig_EISGov_nSetPHi"
  spec_CEngDsT_t/1 -> BC/29  "testSig_CEngDsT_t"
  spec_Oil_tSwmp/1 -> BC/30  "testSig_Oil_tSwmp"
  spec_EngDa_tEng/1 -> BC/31  "testSig_EngDa_tEng"
  spec_EISGov_numCurrFunc/1 -> BC/32  "testSig_EISGov_numCurrFunc"
  spec_EISGov_trqReq/1 -> BC/33  "testSig_EISGov_trqReq"
  spec_Epm_dnEng/1 -> BC/34  "testSig_Epm_dnEng"
  spec_EISGov_trqLosFlt/1 -> BC/35  "testSig_EISGov_trqLosFlt"
  spec_RngMod_trqCrSMin/1 -> BC/36  "testSig_RngMod_trqCrSMin"
  spec_EpmSyn_stSync/1 -> BC/37  "testSig_EpmSyn_stSync"
  spec_CoETS_stTSEATrqSpdReq/1 -> BC/38  "testSig_CoETS_stTSEATrqSpdReq"
  spec_EngDa_tStrt/1 -> BC/39  "testSig_EngDa_tStrt"
  spec_CoEng_tiNormal/1 -> BC/40  "testSig_CoEng_tiNormal"
  spec_EISGov_trqPLo/1 -> BC/41  "testSig_EISGov_trqPLo"
  spec_EISGov_trq/1 -> BC/42  "testSig_EISGov_trq"
  spec_EISGov_trqFlt/1 -> BC/43  "testSig_EISGov_trqFlt"
  spec_SpdGov_trqFlt/1 -> BC/44  "testSig_SpdGov_trqFlt"
  spec_SpdGov_trqSet/1 -> BC/45  "testSig_SpdGov_trqSet"
  spec_SpdGov_trqLead/1 -> BC/46  "testSig_SpdGov_trqLead"

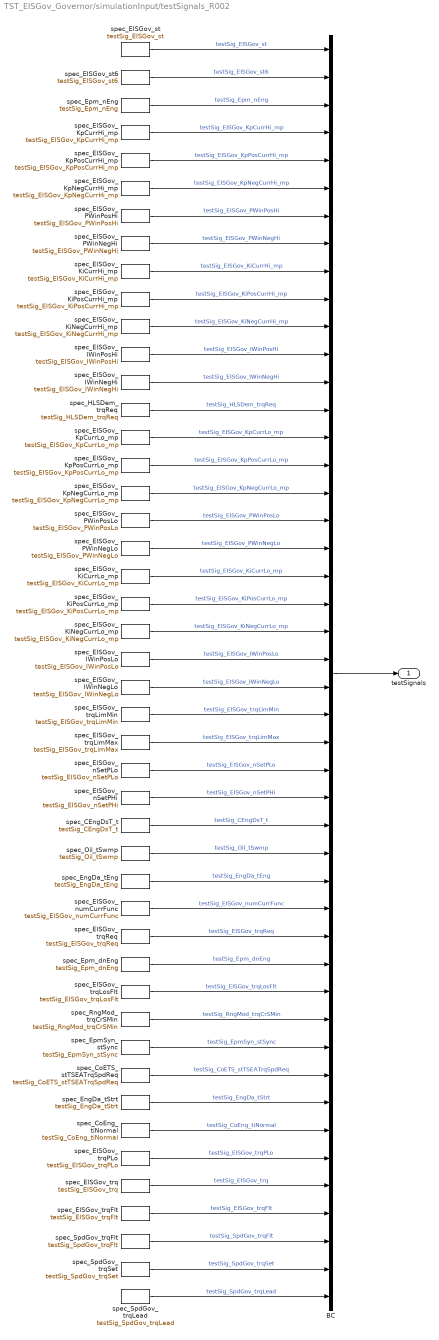
== system TST_EISGov_Governor/simulationInput/testSignals_R002 ==
  BC : BusCreator  Inputs=46
  spec_CEngDsT_t : FromWorkspace  VariableName=testSig_CEngDsT_t  Interpolate=off  OutputAfterFinalValue=Holding final value
  spec_CoETS_stTSEATrqSpdReq : FromWorkspace  VariableName=testSig_CoETS_stTSEATrqSpdReq  Interpolate=off  OutputAfterFinalValue=Holding final value
  spec_CoEng_tiNormal : FromWorkspace  VariableName=testSig_CoEng_tiNormal  Interpolate=off  OutputAfterFinalValue=Holding final value
  spec_EISGov_IWinNegHi : FromWorkspace  VariableName=testSig_EISGov_IWinNegHi  Interpolate=off  OutputAfterFinalValue=Holding final value
  spec_EISGov_IWinNegLo : FromWorkspace  VariableName=testSig_EISGov_IWinNegLo  Interpolate=off  OutputAfterFinalValue=Holding final value
  spec_EISGov_IWinPosHi : FromWorkspace  VariableName=testSig_EISGov_IWinPosHi  Interpolate=off  OutputAfterFinalValue=Holding final value
  spec_EISGov_IWinPosLo : FromWorkspace  VariableName=testSig_EISGov_IWinPosLo  Interpolate=off  OutputAfterFinalValue=Holding final value
  spec_EISGov_KiCurrHi_mp : FromWorkspace  VariableName=testSig_EISGov_KiCurrHi_mp  Interpolate=off  OutputAfterFinalValue=Holding final value
  spec_EISGov_KiCurrLo_mp : FromWorkspace  VariableName=testSig_EISGov_KiCurrLo_mp  Interpolate=off  OutputAfterFinalValue=Holding final value
  spec_EISGov_KiNegCurrHi_mp : FromWorkspace  VariableName=testSig_EISGov_KiNegCurrHi_mp  Interpolate=off  OutputAfterFinalValue=Holding final value
  spec_EISGov_KiNegCurrLo_mp : FromWorkspace  VariableName=testSig_EISGov_KiNegCurrLo_mp  Interpolate=off  OutputAfterFinalValue=Holding final value
  spec_EISGov_KiPosCurrHi_mp : FromWorkspace  VariableName=testSig_EISGov_KiPosCurrHi_mp  Interpolate=off  OutputAfterFinalValue=Holding final value
  spec_EISGov_KiPosCurrLo_mp : FromWorkspace  VariableName=testSig_EISGov_KiPosCurrLo_mp  Interpolate=off  OutputAfterFinalValue=Holding final value
  spec_EISGov_KpCurrHi_mp : FromWorkspace  VariableName=testSig_EISGov_KpCurrHi_mp  Interpolate=off  OutputAfterFinalValue=Holding final value
  spec_EISGov_KpCurrLo_mp : FromWorkspace  VariableName=testSig_EISGov_KpCurrLo_mp  Interpolate=off  OutputAfterFinalValue=Holding final value
  spec_EISGov_KpNegCurrHi_mp : FromWorkspace  VariableName=testSig_EISGov_KpNegCurrHi_mp  Interpolate=off  OutputAfterFinalValue=Holding final value
  spec_EISGov_KpNegCurrLo_mp : FromWorkspace  VariableName=testSig_EISGov_KpNegCurrLo_mp  Interpolate=off  OutputAfterFinalValue=Holding final value
  spec_EISGov_KpPosCurrHi_mp : FromWorkspace  VariableName=testSig_EISGov_KpPosCurrHi_mp  Interpolate=off  OutputAfterFinalValue=Holding final value
  spec_EISGov_KpPosCurrLo_mp : FromWorkspace  VariableName=testSig_EISGov_KpPosCurrLo_mp  Interpolate=off  OutputAfterFinalValue=Holding final value
  spec_EISGov_PWinNegHi : FromWorkspace  VariableName=testSig_EISGov_PWinNegHi  Interpolate=off  OutputAfterFinalValue=Holding final value
  spec_EISGov_PWinNegLo : FromWorkspace  VariableName=testSig_EISGov_PWinNegLo  Interpolate=off  OutputAfterFinalValue=Holding final value
  spec_EISGov_PWinPosHi : FromWorkspace  VariableName=testSig_EISGov_PWinPosHi  Interpolate=off  OutputAfterFinalValue=Holding final value
  spec_EISGov_PWinPosLo : FromWorkspace  VariableName=testSig_EISGov_PWinPosLo  Interpolate=off  OutputAfterFinalValue=Holding final value
  spec_EISGov_nSetPHi : FromWorkspace  VariableName=testSig_EISGov_nSetPHi  Interpolate=off  OutputAfterFinalValue=Holding final value
  spec_EISGov_nSetPLo : FromWorkspace  VariableName=testSig_EISGov_nSetPLo  Interpolate=off  OutputAfterFinalValue=Holding final value
  spec_EISGov_numCurrFunc : FromWorkspace  VariableName=testSig_EISGov_numCurrFunc  Interpolate=off  OutputAfterFinalValue=Holding final value
  spec_EISGov_st : FromWorkspace  VariableName=testSig_EISGov_st  Interpolate=off  OutputAfterFinalValue=Holding final value
  spec_EISGov_st6 : FromWorkspace  VariableName=testSig_EISGov_st6  Interpolate=off  OutputAfterFinalValue=Holding final value
  spec_EISGov_trq : FromWorkspace  VariableName=testSig_EISGov_trq  Interpolate=off  OutputAfterFinalValue=Holding final value
  spec_EISGov_trqFlt : FromWorkspace  VariableName=testSig_EISGov_trqFlt  Interpolate=off  OutputAfterFinalValue=Holding final value
  spec_EISGov_trqLimMax : FromWorkspace  VariableName=testSig_EISGov_trqLimMax  Interpolate=off  OutputAfterFinalValue=Holding final value
  spec_EISGov_trqLimMin : FromWorkspace  VariableName=testSig_EISGov_trqLimMin  Interpolate=off  OutputAfterFinalValue=Holding final value
  spec_EISGov_trqLosFlt : FromWorkspace  VariableName=testSig_EISGov_trqLosFlt  Interpolate=off  OutputAfterFinalValue=Holding final value
  spec_EISGov_trqPLo : FromWorkspace  VariableName=testSig_EISGov_trqPLo  Interpolate=off  OutputAfterFinalValue=Holding final value
  spec_EISGov_trqReq : FromWorkspace  VariableName=testSig_EISGov_trqReq  Interpolate=off  OutputAfterFinalValue=Holding final value
  spec_EngDa_tEng : FromWorkspace  VariableName=testSig_EngDa_tEng  Interpolate=off  OutputAfterFinalValue=Holding final value
  spec_EngDa_tStrt : FromWorkspace  VariableName=testSig_EngDa_tStrt  Interpolate=off  OutputAfterFinalValue=Holding final value
  spec_EpmSyn_stSync : FromWorkspace  VariableName=testSig_EpmSyn_stSync  Interpolate=off  OutputAfterFinalValue=Holding final value
  spec_Epm_dnEng : FromWorkspace  VariableName=testSig_Epm_dnEng  Interpolate=off  OutputAfterFinalValue=Holding final value
  spec_Epm_nEng : FromWorkspace  VariableName=testSig_Epm_nEng  Interpolate=off  OutputAfterFinalValue=Holding final value
  spec_HLSDem_trqReq : FromWorkspace  VariableName=testSig_HLSDem_trqReq  Interpolate=off  OutputAfterFinalValue=Holding final value
  spec_Oil_tSwmp : FromWorkspace  VariableName=testSig_Oil_tSwmp  Interpolate=off  OutputAfterFinalValue=Holding final value
  spec_RngMod_trqCrSMin : FromWorkspace  VariableName=testSig_RngMod_trqCrSMin  Interpolate=off  OutputAfterFinalValue=Holding final value
  spec_SpdGov_trqFlt : FromWorkspace  VariableName=testSig_SpdGov_trqFlt  Interpolate=off  OutputAfterFinalValue=Holding final value
  spec_SpdGov_trqLead : FromWorkspace  VariableName=testSig_SpdGov_trqLead  Interpolate=off  OutputAfterFinalValue=Holding final value
  spec_SpdGov_trqSet : FromWorkspace  VariableName=testSig_SpdGov_trqSet  Interpolate=off  OutputAfterFinalValue=Holding final value
  testSignals : Outport
  wires:
  BC/1 -> testSignals/1
  spec_EISGov_st/1 -> BC/1  "testSig_EISGov_st"
  spec_EISGov_st6/1 -> BC/2  "testSig_EISGov_st6"
  spec_Epm_nEng/1 -> BC/3  "testSig_Epm_nEng"
  spec_EISGov_KpCurrHi_mp/1 -> BC/4  "testSig_EISGov_KpCurrHi_mp"
  spec_EISGov_KpPosCurrHi_mp/1 -> BC/5  "testSig_EISGov_KpPosCurrHi_mp"
  spec_EISGov_KpNegCurrHi_mp/1 -> BC/6  "testSig_EISGov_KpNegCurrHi_mp"
  spec_EISGov_PWinPosHi/1 -> BC/7  "testSig_EISGov_PWinPosHi"
  spec_EISGov_PWinNegHi/1 -> BC/8  "testSig_EISGov_PWinNegHi"
  spec_EISGov_KiCurrHi_mp/1 -> BC/9  "testSig_EISGov_KiCurrHi_mp"
  spec_EISGov_KiPosCurrHi_mp/1 -> BC/10  "testSig_EISGov_KiPosCurrHi_mp"
  spec_EISGov_KiNegCurrHi_mp/1 -> BC/11  "testSig_EISGov_KiNegCurrHi_mp"
  spec_EISGov_IWinPosHi/1 -> BC/12  "testSig_EISGov_IWinPosHi"
  spec_EISGov_IWinNegHi/1 -> BC/13  "testSig_EISGov_IWinNegHi"
  spec_HLSDem_trqReq/1 -> BC/14  "testSig_HLSDem_trqReq"
  spec_EISGov_KpCurrLo_mp/1 -> BC/15  "testSig_EISGov_KpCurrLo_mp"
  spec_EISGov_KpPosCurrLo_mp/1 -> BC/16  "testSig_EISGov_KpPosCurrLo_mp"
  spec_EISGov_KpNegCurrLo_mp/1 -> BC/17  "testSig_EISGov_KpNegCurrLo_mp"
  spec_EISGov_PWinPosLo/1 -> BC/18  "testSig_EISGov_PWinPosLo"
  spec_EISGov_PWinNegLo/1 -> BC/19  "testSig_EISGov_PWinNegLo"
  spec_EISGov_KiCurrLo_mp/1 -> BC/20  "testSig_EISGov_KiCurrLo_mp"
  spec_EISGov_KiPosCurrLo_mp/1 -> BC/21  "testSig_EISGov_KiPosCurrLo_mp"
  spec_EISGov_KiNegCurrLo_mp/1 -> BC/22  "testSig_EISGov_KiNegCurrLo_mp"
  spec_EISGov_IWinPosLo/1 -> BC/23  "testSig_EISGov_IWinPosLo"
  spec_EISGov_IWinNegLo/1 -> BC/24  "testSig_EISGov_IWinNegLo"
  spec_EISGov_trqLimMin/1 -> BC/25  "testSig_EISGov_trqLimMin"
  spec_EISGov_trqLimMax/1 -> BC/26  "testSig_EISGov_trqLimMax"
  spec_EISGov_nSetPLo/1 -> BC/27  "testSig_EISGov_nSetPLo"
  spec_EISGov_nSetPHi/1 -> BC/28  "testSig_EISGov_nSetPHi"
  spec_CEngDsT_t/1 -> BC/29  "testSig_CEngDsT_t"
  spec_Oil_tSwmp/1 -> BC/30  "testSig_Oil_tSwmp"
  spec_EngDa_tEng/1 -> BC/31  "testSig_EngDa_tEng"
  spec_EISGov_numCurrFunc/1 -> BC/32  "testSig_EISGov_numCurrFunc"
  spec_EISGov_trqReq/1 -> BC/33  "testSig_EISGov_trqReq"
  spec_Epm_dnEng/1 -> BC/34  "testSig_Epm_dnEng"
  spec_EISGov_trqLosFlt/1 -> BC/35  "testSig_EISGov_trqLosFlt"
  spec_RngMod_trqCrSMin/1 -> BC/36  "testSig_RngMod_trqCrSMin"
  spec_EpmSyn_stSync/1 -> BC/37  "testSig_EpmSyn_stSync"
  spec_CoETS_stTSEATrqSpdReq/1 -> BC/38  "testSig_CoETS_stTSEATrqSpdReq"
  spec_EngDa_tStrt/1 -> BC/39  "testSig_EngDa_tStrt"
  spec_CoEng_tiNormal/1 -> BC/40  "testSig_CoEng_tiNormal"
  spec_EISGov_trqPLo/1 -> BC/41  "testSig_EISGov_trqPLo"
  spec_EISGov_trq/1 -> BC/42  "testSig_EISGov_trq"
  spec_EISGov_trqFlt/1 -> BC/43  "testSig_EISGov_trqFlt"
  spec_SpdGov_trqFlt/1 -> BC/44  "testSig_SpdGov_trqFlt"
  spec_SpdGov_trqSet/1 -> BC/45  "testSig_SpdGov_trqSet"
  spec_SpdGov_trqLead/1 -> BC/46  "testSig_SpdGov_trqLead"
